simulink model "logical_unit"  (R2022a)
settings: Solver=VariableStepAuto  StartTime=0.0  StopTime=10.0  RelTol=1e-3
settings Model: Creator=cuomo  LastModifiedBy=cuomo

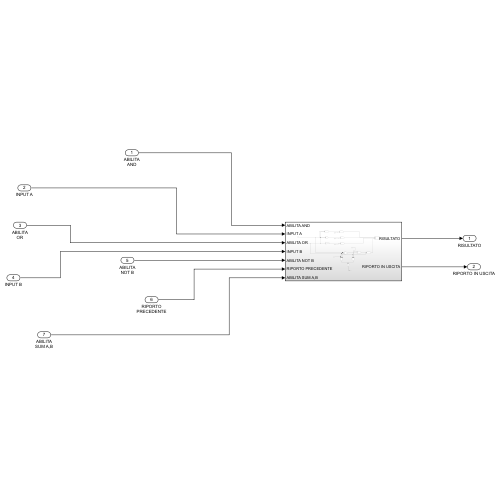
[thumbnail: Simulink's stored preview of the top-level diagram]
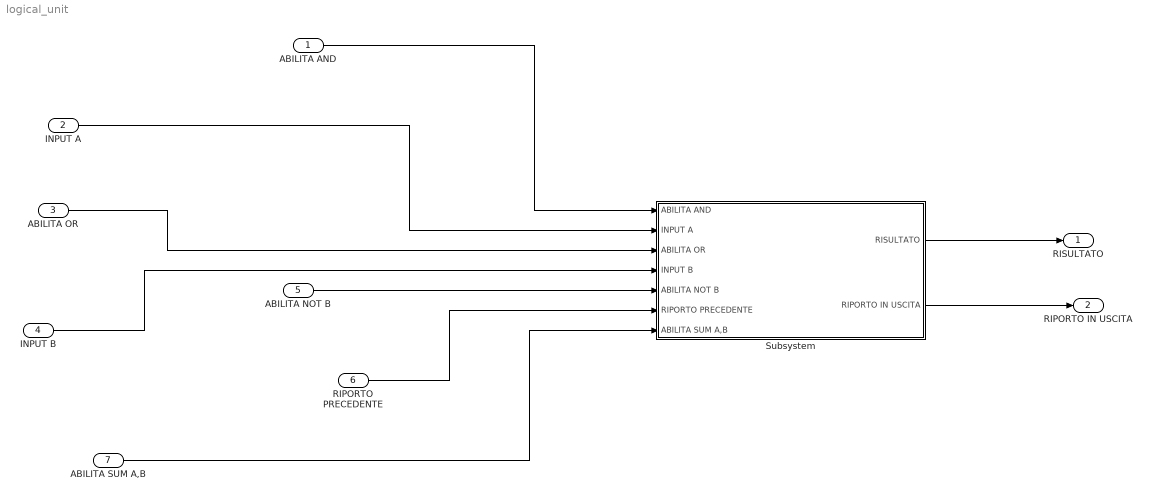
== system logical_unit ==
  ABILITA AND : Inport
  INPUT A : Inport  Port=2
  ABILITA OR : Inport  Port=3
  INPUT B : Inport  Port=4
  ABILITA NOT B : Inport  Port=5
  RIPORTO PRECEDENTE : Inport  Port=6
  ABILITA SUM A,B : Inport  Port=7
  Subsystem : Subsystem
  RISULTATO : Outport
  RIPORTO IN USCITA : Outport  Port=2
  wires:
  ABILITA AND/1 -> Subsystem/1(ABILITA AND)
  INPUT A/1 -> Subsystem/2(INPUT A)
  ABILITA OR/1 -> Subsystem/3(ABILITA OR)
  INPUT B/1 -> Subsystem/4(INPUT B)
  ABILITA NOT B/1 -> Subsystem/5(ABILITA NOT B)
  RIPORTO PRECEDENTE/1 -> Subsystem/6(RIPORTO PRECEDENTE)
  ABILITA SUM A,B/1 -> Subsystem/7(ABILITA SUM A,B)
  Subsystem/1(RISULTATO) -> RISULTATO/1
  Subsystem/2(RIPORTO IN USCITA) -> RIPORTO IN USCITA/1

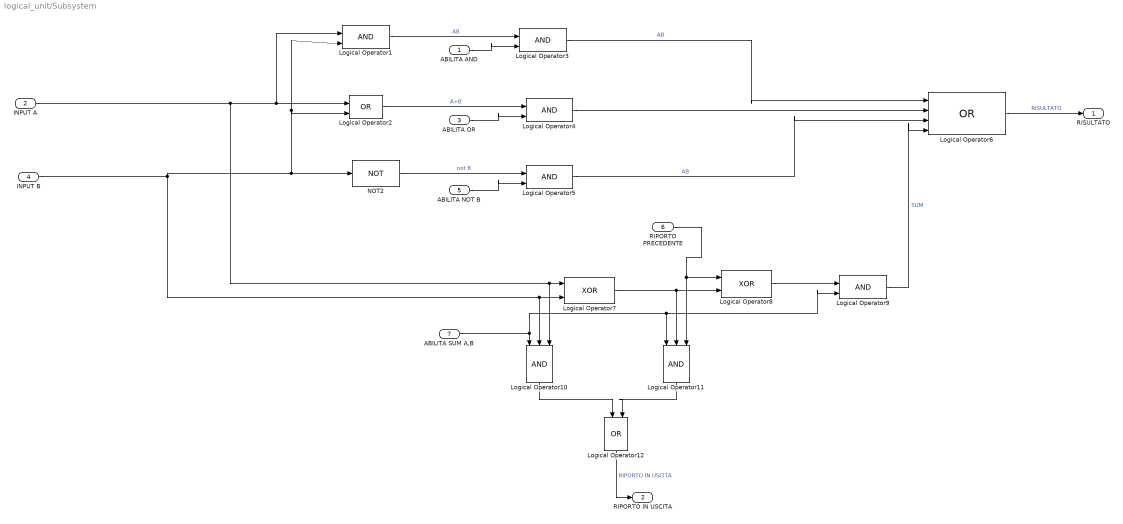
== system logical_unit/Subsystem ==
  ABILITA AND : Inport
  INPUT A : Inport  Port=2
  ABILITA OR : Inport  Port=3
  INPUT B : Inport  Port=4
  ABILITA NOT B : Inport  Port=5
  RIPORTO PRECEDENTE : Inport  Port=6
  ABILITA SUM A,B : Inport  Port=7
  Logical Operator{1,3..5,9} (5 alike) : Logic  IconShape=distinctive  AllPortsSameDT=off  OutDataTypeStr=boolean
  Logical Operator10 : Logic  Inputs=3  IconShape=distinctive  AllPortsSameDT=off  OutDataTypeStr=boolean
  Logical Operator11 : Logic  Inputs=3  IconShape=distinctive  AllPortsSameDT=off  OutDataTypeStr=boolean
  Logical Operator12 : Logic  Operator=OR  IconShape=distinctive  AllPortsSameDT=off  OutDataTypeStr=boolean
  Logical Operator2 : Logic  Operator=OR  IconShape=distinctive  AllPortsSameDT=off  OutDataTypeStr=boolean
  Logical Operator6 : Logic  Operator=OR  Inputs=4  IconShape=distinctive  AllPortsSameDT=off  OutDataTypeStr=boolean
  Logical Operator7 : Logic  Operator=XOR  IconShape=distinctive  AllPortsSameDT=off  OutDataTypeStr=boolean
  Logical Operator8 : Logic  Operator=XOR  IconShape=distinctive  AllPortsSameDT=off  OutDataTypeStr=boolean
  NOT2 : Logic  Operator=NOT  IconShape=distinctive  AllPortsSameDT=off  OutDataTypeStr=boolean
  RISULTATO : Outport
  RIPORTO IN USCITA : Outport  Port=2
  wires:
  ABILITA AND/1 -> Logical Operator3/2
  Logical Operator7/1 -> Logical Operator11/2, Logical Operator8/2
  RIPORTO PRECEDENTE/1 -> Logical Operator8/1, Logical Operator11/3
  Logical Operator12/1 -> RIPORTO IN USCITA/1  "RIPORTO IN USCITA"
  NOT2/1 -> Logical Operator5/1  "not B"
  Logical Operator3/1 -> Logical Operator6/1  "AB"
  Logical Operator5/1 -> Logical Operator6/3  "AB"
  INPUT A/1 -> Logical Operator1/1, Logical Operator2/1, Logical Operator10/3, Logical Operator7/1
  INPUT B/1 -> Logical Operator1/2, Logical Operator2/2, NOT2/1, Logical Operator10/2, Logical Operator7/2
  Logical Operator2/1 -> Logical Operator4/1  "A+B"
  ABILITA SUM A,B/1 -> Logical Operator11/1, Logical Operator9/2, Logical Operator10/1
  Logical Operator9/1 -> Logical Operator6/4  "SUM"
  ABILITA NOT B/1 -> Logical Operator5/2
  Logical Operator11/1 -> Logical Operator12/2
  Logical Operator10/1 -> Logical Operator12/1
  ABILITA OR/1 -> Logical Operator4/2
  Logical Operator8/1 -> Logical Operator9/1
  Logical Operator6/1 -> RISULTATO/1  "RISULTATO"
  Logical Operator1/1 -> Logical Operator3/1  "AB"
  Logical Operator4/1 -> Logical Operator6/2
